simulink model "primerModeloStateflow"  (R2017a)
settings: Solver=VariableStepAuto  StartTime=0.0  StopTime=10.0  RelTol=1e-3
InitFcn:
  | algunasConstantes
settings Model: Creator=yellow submarine  LastModifiedBy=yellow submarine

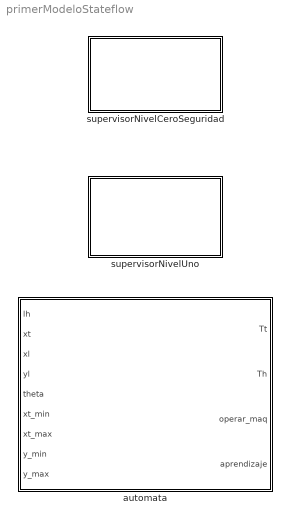
== system primerModeloStateflow ==
  automata : Stateflow chart  TreatAsAtomicUnit=on
  supervisorNivelCeroSeguridad : Stateflow chart  TreatAsAtomicUnit=on
  supervisorNivelUno : Stateflow chart  TreatAsAtomicUnit=on

== stateflow chart primerModeloStateflow/supervisorNivelUno ==
  state verificaLimitesCarro
    during: verificaLimitesXt();
  state verificaAlturaGancho
    during: verificaLimitesGancho();
  function verificaLimitesXt:
    | function verificaLimitesXt
    | 
    | if xt>xt_max || xt<=xt_min
    |     paradaDeEmergencia=1;
    | end
    |  
    | end
  function verificaLimitesGancho:
    | function verificaLimitesGancho
    | 
    | if l>y_max || l<=y_min
    |     paradaDeEmergencia=1;
    | end
    |  
    | end

== stateflow chart primerModeloStateflow/supervisorNivelCeroSeguridad ==

== stateflow chart primerModeloStateflow/automata ==
  state maquinaEncendida
    state operacionDeLaMaquina [parallel]
      settings: executionOrder=1
      state operacionNormal
        state maquinaEnoperacion
          state modoOperacionManual
          state modoOperacionAutomatica
          state transfiriendoModoDeOperacion
          (default) -> modoOperacionManual
          modoOperacionAutomatica -> modoOperacionManual
          modoOperacionManual -> transfiriendoModoDeOperacion
          transfiriendoModoDeOperacion -> modoOperacionAutomatica
        state inicio
        state configuracion
        maquinaEnoperacion -> inicio : {operar_maq=0}
        inicio -> maquinaEnoperacion [order 1] : {operar_maq=1}
        (default) -> inicio
        inicio -> configuracion [order 2] : {aprendizaje=1}
        configuracion -> inicio : {aprendizaje=0}
      state operacionEmergencia
        entry:
        Tt=0
        Th=0
      (default) -> operacionNormal
      operacionNormal -> operacionEmergencia : [lh>=lx_max]
    state gancho [parallel]
      settings: executionOrder=2
  data: lh input; lx_max constant double; xt input; xl input; yl input; theta input; Tt output; Th output; operar_maq output; aprendizaje output; xt_min input; xt_max input; y_min input; y_max input
